simulink model "Quadcopter_LQR_3DOF"  (R2022a)
settings: Solver=VariableStepAuto  StartTime=0.0  StopTime=10.0  RelTol=1e-3
undefined symbols (not defined in the file): A, B, C, Klqr
settings Model: Creator=creec  LastModifiedBy=creec

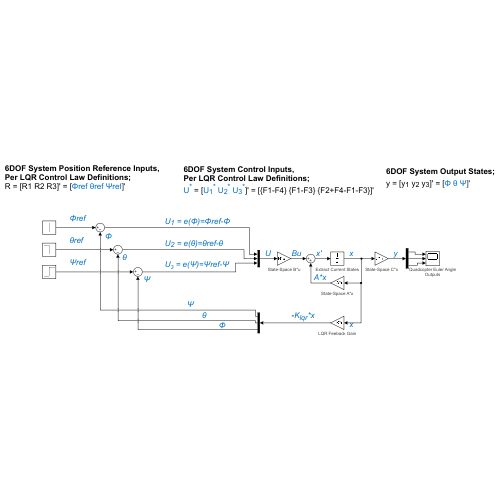
[thumbnail: Simulink's stored preview of the top-level diagram]
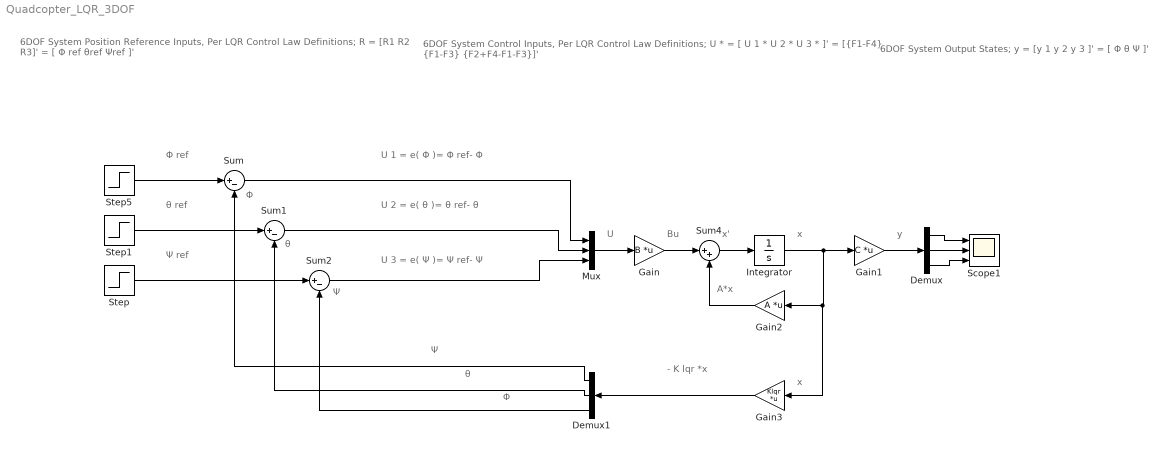
== system Quadcopter_LQR_3DOF ==
  note: θ
  note: θ ref
  note: Ψ
  note: 6DOF System Control Inputs,
      | Per LQR Control Law Definitions;
      | U * = [ U 1 * U 2 * U 3 * ]' = [{F1-F4} {F1-F3} {F2+F4-F1-F3}]'
  note: - K lqr *x
  note: Ψ
  note: 6DOF System Output States;
      | y = [y 1 y 2 y 3 ]' = [ Φ θ Ψ ]'
  note: x'
  note: U 3 = e( Ψ )= Ψ ref- Ψ
  note: Φ
  note: 6DOF System Position Reference Inputs,
      | Per LQR Control Law Definitions;
      | R = [R1 R2 R3]' = [ Φ ref θref Ψref ]'
  note: U 2 = e( θ )= θ ref- θ
  note: U 1 = e( Φ )= Φ ref- Φ
  note: θ
  note: Φ
  note: x
  note: A*x
  note: y
  note: Ψ ref
  note: Φ ref
  note: x
  note: Bu
  note: U
  Demux : Demux  Outputs=3
  Demux1 : Demux  Outputs=3
  Gain : Gain  Gain=B  Multiplication=Matrix(K*u)
      settings: AttributesFormatString=State-Space B*u
  Gain1 : Gain  Gain=C  Multiplication=Matrix(K*u)
      settings: AttributesFormatString=State-Space C*x
  Gain2 : Gain  Gain=A  Multiplication=Matrix(K*u)
      settings: AttributesFormatString=State-Space A*x
  Gain3 : Gain  Gain=Klqr  Multiplication=Matrix(K*u)
      settings: AttributesFormatString=LQR Feeback Gain
  Integrator : Integrator
      settings: AttributesFormatString=Extract Current States
  Mux : Mux  Inputs=3
  Scope1 : Scope  NumInputPorts=3
      settings: AttributesFormatString=|
      | Quadcopter Euler Angle
      | Outputs
  Step : Step  After=1.5  SampleTime=0
  Step1 : Step  After=-2  SampleTime=0
  Step5 : Step  SampleTime=0
  Sum : Sum  Inputs=|+-
  Sum1 : Sum  Inputs=|+-
  Sum2 : Sum  Inputs=|+-
  Sum4 : Sum  Inputs=|++
  wires:
  Sum2/1 -> Mux/3
  Sum4/1 -> Integrator/1
  Sum/1 -> Mux/1
  Demux1/3 -> Sum2/2
  Step1/1 -> Sum1/1
  Gain3/1 -> Demux1/1
  Demux1/2 -> Sum1/2
  Sum1/1 -> Mux/2
  Step5/1 -> Sum/1
  Step/1 -> Sum2/1
  Gain1/1 -> Demux/1
  Gain2/1 -> Sum4/2
  Gain/1 -> Sum4/1
  Integrator/1 -> Gain1/1, Gain3/1, Gain2/1
  Mux/1 -> Gain/1
  Demux1/1 -> Sum/2
  Demux/1 -> Scope1/1
  Demux/2 -> Scope1/2
  Demux/3 -> Scope1/3
